simulink model "simcape_real_time_V2"  (R2022b)
settings: Solver=ode8  StartTime=0.0  StopTime=100  FixedStep=0.002  RelTol=1e-3
undefined symbols (not defined in the file): drone_leg, K_LQR, K_LQR_GOC, pitch_init, roll_init, v_pitch_init, v_roll_init, v_x_init, v_y_init, v_yaw_init, v_z_init, X, x_init, Y, y_init, yaw_init, Z, z_init
libraries: sm_lib x55, nesl_utility x12, simulink x7
(part 1 of 3)
settings Model: Creator=tridu  LastModifiedBy=tanda

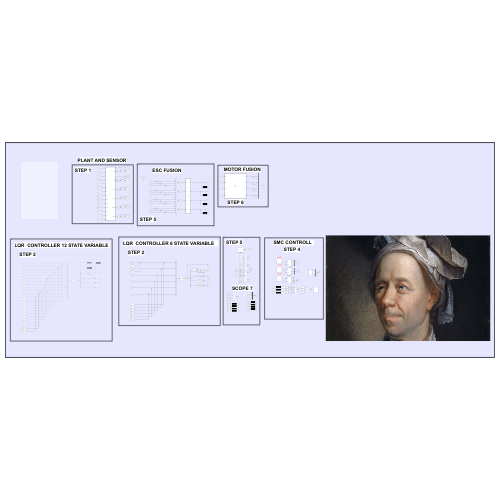
[thumbnail: Simulink's stored preview of the top-level diagram]
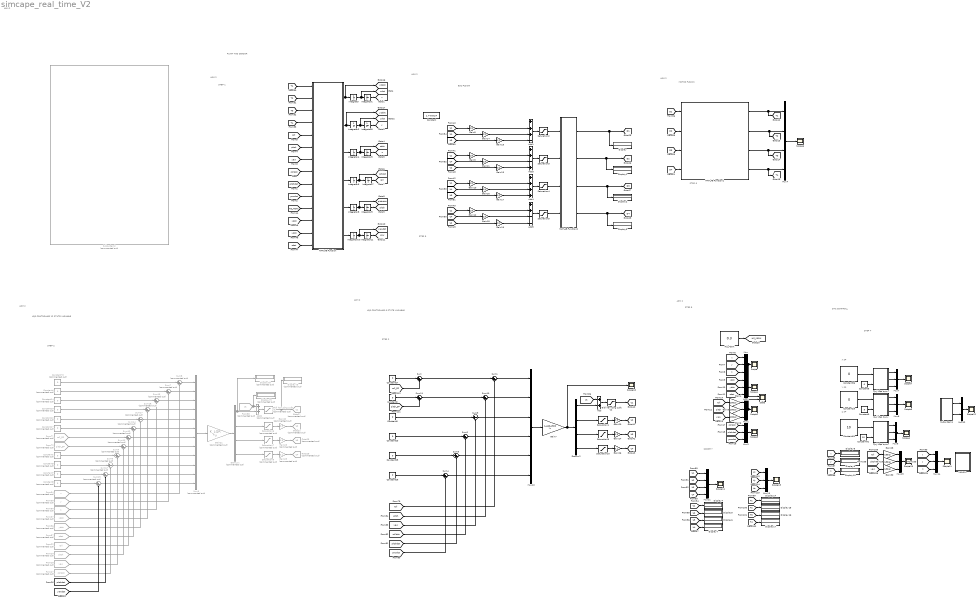
== system simcape_real_time_V2 ==
  note: ARM 2
  note: STEP 5
  note: SCOPE 7
  note: ARM 2
  note: STEP 5
  note: STEP 1
  note: ARM 2
  note: STEP 6
  note: PLANT AND SENSOR
  note: LQR CONTROLLER 12 STATE VARIABLE
  note: STEP 2
  note: ARM 2
  note: STEP 4
  note: X SP
  note: MOTOR FUSION
  note: ARM 2
  note: STEP 2
  note: Y SP
  note: ARM 2
  note: ESC FUSION
  note: Z SP
  note: SMC CONTROLL
  note: ARM 2
  note: LQR CONTROLLER 6 STATE VARIABLE
  Add : Sum
  Add1 : Sum  Inputs=+++-
  Add2 : Sum  Commented=on
  Add3 : Sum  Inputs=++-+
  Add4 : Sum  Inputs=++++
  Add5 : Sum  Inputs=++--
  Constant : Constant  Value=1.7*9.81/4
  Constant{1,4..5,7..8,13..17} (10 alike) : Constant  Commented=on  Value=0
  Constant{2..3,6,23,25..27,29,36} (9 alike) : Constant  Value=0
  Constant31 : Constant  Value=10
  Constant42 : Constant  Value=10
  Constant9 : Constant  Value=5
  Demux1 : Demux  Commented=on
  Demux2 : Demux
  Display{,1..10,14..17} (15 alike) : Display
  Display13 : Display  Commented=on
  Display18 : Display  Commented=on
  Display19 : Display  Commented=on
  From22 : From  Commented=on  GotoTag=roll  TagVisibility=global
  From27 : From  Commented=on  GotoTag=rolldot  TagVisibility=global
  From28 : From  Commented=on  GotoTag=yaw  TagVisibility=global
  From29 : From  Commented=on  GotoTag=pitch  TagVisibility=global
  From34 : From  Commented=on  GotoTag=x  TagVisibility=global
  From35 : From  Commented=on  GotoTag=y  TagVisibility=global
  From36 : From  Commented=on  GotoTag=ydot  TagVisibility=global
  From37 : From  Commented=on  GotoTag=xdot  TagVisibility=global
  From38 : From  Commented=on  GotoTag=Uz  TagVisibility=global
  From57 : From  Commented=on  GotoTag=zdot  TagVisibility=global
  From60 : From  Commented=on  GotoTag=z  TagVisibility=global
  From71 : From  Commented=on  GotoTag=roll_SP  TagVisibility=global
  From72 : From  Commented=on  GotoTag=pitch_SP  TagVisibility=global
  Gain{8..12,14,16,18} (8 alike) : Gain  Gain=1/4
  Gain{13,15,17,19} (4 alike) : Gain  Gain=1/2
  Gain20 : Gain  Gain=0.3
  Gain21 : Gain  Commented=on  Gain=K_LQR  Multiplication=Matrix(K*u)
  Gain22 : Gain  Commented=on  Gain=0.3
  Gain23 : Gain  Commented=on  Gain=0.3
  Gain24 : Gain  Gain=0.3
  Gain25 : Gain  Commented=on  Gain=0.1
  Gain26 : Gain  Gain=0.1
  Gain{4..6,28..30} (6 alike) : Gain  Gain=180/pi
  Gain7 : Gain  Gain=K_LQR_GOC  Multiplication=Matrix(K*u)
  Giới hạn công suất U1 : Saturate  Commented=on  UpperLimit=29.3230*0.3  LowerLimit=-1.7*9.81
  Giới hạn công suất U2 : Saturate  UpperLimit=25  LowerLimit=-1.7*9.81
  Goto21 : Goto  Commented=on  GotoTag=U1  TagVisibility=global
  Goto22 : Goto  Commented=on  GotoTag=U2  TagVisibility=global
  Goto23 : Goto  Commented=on  GotoTag=U3  TagVisibility=global
  Goto29 : Goto  Commented=on  GotoTag=U4  TagVisibility=global
  HS_MSKK : Constant  Value=0.3
  Integrator : Integrator  InitialCondition=v_x_init
  Integrator1 : Integrator  InitialCondition=x_init
  Integrator10 : Integrator  InitialCondition=v_yaw_init
  Integrator11 : Integrator  InitialCondition=yaw_init
  Integrator2 : Integrator  InitialCondition=v_y_init
  Integrator3 : Integrator  InitialCondition=y_init
  Integrator4 : Integrator  InitialCondition=z_init
  Integrator5 : Integrator  InitialCondition=v_z_init
  Integrator6 : Integrator  InitialCondition=v_roll_init
  Integrator7 : Integrator  InitialCondition=roll_init
  Integrator8 : Integrator  InitialCondition=v_pitch_init
  Integrator9 : Integrator  InitialCondition=pitch_init
  MATLAB Function : MATLAB Function  TreatAsAtomicUnit=on
  MATLAB Function1 : MATLAB Function  TreatAsAtomicUnit=on
  MATLAB Function2 : MATLAB Function  TreatAsAtomicUnit=on
  MOVE L : Subsystem
  Mux{,1..3,6..8,13..15} (10 alike) : Mux  Inputs=3
  Mux10 : Mux  Inputs=6
  Mux11 : Mux
  Mux12 : Mux  Inputs=2
  Mux4 : Mux
  Mux5 : Mux  Commented=on  Inputs=12
  Quỹ đạo trục x : Subsystem
  Quỹ đạo trục y : Subsystem
  Quỹ đạo trục z : Subsystem
  Saturation1 : Saturate  UpperLimit=11.5  LowerLimit=-11.5
  Saturation10 : Saturate  UpperLimit=11.5+11.5  LowerLimit=-23
  Saturation{2..5} (4 alike) : Saturate  UpperLimit=11.5  LowerLimit=0
  Saturation6 : Saturate  Commented=on  UpperLimit=11.5  LowerLimit=-11.5
  Saturation7 : Saturate  Commented=on  UpperLimit=11.5  LowerLimit=-11.5
  Saturation8 : Saturate  UpperLimit=11.5  LowerLimit=-11.5
  Saturation9 : Saturate  Commented=on  UpperLimit=11.5  LowerLimit=-11.5
  Scope{,1..4,6..8,10..15} (14 alike) : Scope
  State : Scope  NumInputPorts=2
  Subsystem2 : Subsystem  Commented=on
  Subsystem4 : Subsystem
  Sum : Sum  Inputs=|++
  Sum{1..4,9..10} (6 alike) : Sum  Inputs=|+-
  Sum11 : Sum  Inputs=|++
  Sum{5..8,12..19} (12 alike) : Sum  Commented=on  Inputs=|+-
  tag scope: D1=global, D2=global, D3=global, D4=global, HS_MSKK=global, T1=global, T2=global, T3=global, T4=global, U1=global, U2=global, U3=global, U4=global, pitch=global, pitchdot=global, roll=global, rolldot=global, x2dot=global, x=global, xdot=global, y2dot=global, y=global, yaw=global, yawdot=global, ydot=global, z=global, zdot=global
  wires:
  [pitchdot] -> Mux3/2
  MATLAB Function/3(z2dot) -> Integrator4/1
  Integrator3/1 -> [y]
  Integrator4/1 -> [zdot], Integrator5/1
  Mux1/1 -> Scope1/1
  Integrator7/1 -> [roll]
  [pitchdot] -> MATLAB Function/9(pitch_dot)
  [T3] -> MATLAB Function/3(T3)
  Add5/1 -> Saturation5/1
  MATLAB Function/2(y2dot) -> [y2dot], Integrator2/1
  Mux7/1 -> Scope7/1
  [roll] -> Sum1/2
  [ydot] -> MATLAB Function/13(y_dot)
  Subsystem4/2(Pitch SP) -> Mux12/2
  MATLAB Function1/1(T1) -> Mux4/1, [T1]
  Gain15/1 -> Add1/4
  [roll] -> MATLAB Function/5(roll)
  Mux8/1 -> Scope8/1
  [rolldot] -> Mux3/1
  Integrator11/1 -> [yaw]
  Gain10/1 -> Add4/2
  Giới hạn công suất U2/1 -> [U1]
  Sum2/1 -> Mux10/4
  Mux6/1 -> Scope4/1
  Quỹ đạo trục y/1(X_y) -> Mux8/1
  Quỹ đạo trục z/1(X_z) -> Mux6/1
  Quỹ đạo trục z/2(V_z) -> Mux6/2
  Constant9/1 -> Quỹ đạo trục y/2(v_qd_y)
  Add/1 -> Giới hạn công suất U2/1
  Quỹ đạo trục z/3(A_z) -> Mux6/3
  [HS_MSKK] -> MATLAB Function/11(HS_MSKK)
  Subsystem4/1(Roll SP) -> Mux12/1
  Quỹ đạo trục x/1(X_x) -> Mux7/1
  [pitch_SP] -> Sum11/2
  Mux15/1 -> Scope15/1
  Mux14/1 -> Scope14/1
  [T3] -> Display16/1
  Mux11/1 -> Scope11/1
  [U4] -> Gain16/1
  Integrator9/1 -> [pitch]
  [y] -> Mux14/2
  [U1] -> Gain12/1
  Gain5/1 -> Mux2/2
  Sum17/1 -> Mux5/5
  Quỹ đạo trục x/3(A_x) -> Mux7/3
  [U1] -> Gain8/1
  Gain25/1 -> Goto29/1
  Gain24/1 -> [U3]
  [rolldot] -> Sum2/2
  Integrator8/1 -> [pitchdot], Integrator9/1
  Quỹ đạo trục y/3(A_y) -> Mux8/3
  Mux2/1 -> State/2, Scope2/1
  [pitch] -> Sum10/2
  [zdot] -> Mux1/3
  Constant13/1 -> Sum8/1
  [pitch] -> Gain29/1
  [yaw] -> Gain30/1
  Gain12/1 -> Add5/2
  Demux2/2 -> Saturation1/1
  [yawdot] -> Sum4/2
  Sum14/1 -> Mux5/6
  Gain30/1 -> Mux15/3
  [Ux] -> Mux13/1
  [z] -> Mux14/3
  Mux13/1 -> Scope13/1
  MATLAB Function2/3(D3) -> Display2/1, [D3]
  Sum11/1 -> Sum10/1
  [T4] -> Display17/1
  [yaw] -> Sum9/2
  [roll_SP] -> Sum/2
  Mux10/1 -> Gain7/1
  [x] -> Display8/1
  [D3] -> MATLAB Function1/3(D3)
  Gain20/1 -> [U2]
  [T2] -> Display15/1
  [zdot] -> MATLAB Function/14(z_dot)
  Quỹ đạo trục y/2(V_y) -> Mux8/2
  [Uz] -> Add/1
  [T1] -> Display14/1
  Integrator5/1 -> [z]
  [U3] -> Display6/1
  Giới hạn công suất U1/1 -> Display13/1, Goto21/1
  [D4] -> MATLAB Function1/4(D4)
  [U1] -> Display4/1
  Sum4/1 -> Mux10/6
  [yaw] -> MATLAB Function/7(yaw)
  Gain9/1 -> Add3/2
  Gain4/1 -> Mux2/1
  [U3] -> Mux11/3
  [U1] -> Mux11/1
  [x] -> Mux14/1
  [U2] -> Mux11/2
  MATLAB Function/5(pitch2dot) -> Integrator8/1
  [pitch] -> Gain5/1
  Mux5/1 -> Gain21/1
  [U1] -> Gain9/1
  [Uz] -> Mux13/3
  [U4] -> Gain11/1
  Gain8/1 -> Add1/2
  Gain23/1 -> Goto23/1
  Sum10/1 -> Mux10/2
  Sum9/1 -> Mux10/3
  Gain17/1 -> Add4/4
  Gain6/1 -> Mux2/3
  Integrator10/1 -> [yawdot], Integrator11/1
  Demux1/3 -> Saturation7/1
  Sum3/1 -> Mux10/5
  Mux3/1 -> Scope3/1
  Gain7/1 -> Demux2/1, Scope10/1
  Constant26/1 -> Sum4/1
  [pitch] -> MATLAB Function/6(pitch)
  [U4] -> Mux11/4
  Constant23/1 -> Sum2/1
  Sum15/1 -> Mux5/7
  Constant4/1 -> Sum7/1
  Integrator2/1 -> [ydot], Integrator3/1
  [xdot] -> Mux1/1
  [U2] -> Gain13/1
  [U1] -> Gain10/1
  Quỹ đạo trục x/2(V_x) -> Mux7/2
  Add3/1 -> Saturation3/1
  [xdot] -> MATLAB Function/12(x_dot)
  Add1/1 -> Saturation2/1
  [T1] -> MATLAB Function/1(T1)
  [y] -> Mux/2
  Constant25/1 -> Sum3/1
  Constant6/1 -> Quỹ đạo trục x/2(v_qd_x)
  Mux/1 -> State/1, Scope/1
  Saturation1/1 -> Gain20/1
  [yawdot] -> Mux3/3
  [T4] -> MATLAB Function/4(T4)
  [yawdot] -> MATLAB Function/10(yaw_dot)
  [Uy] -> Mux13/2
  Gain26/1 -> [U4]
  MATLAB Function/1(x2dot) -> [x2dot], Integrator/1
  Saturation3/1 -> MATLAB Function2/2(T2)
  Demux2/3 -> Saturation8/1
  Demux2/4 -> Saturation10/1
  [pitchdot] -> Sum3/2
  Mux12/1 -> Scope12/1
  Gain28/1 -> Mux15/1
  [T2] -> MATLAB Function/2(T2)
  Constant3/1 -> Sum9/1
  Sum1/1 -> Mux10/1
  Sum8/1 -> Mux5/1
  Saturation5/1 -> MATLAB Function2/4(T4)
  [D1] -> MATLAB Function1/1(D1)
  [D2] -> MATLAB Function1/2(D2)
  [z] -> Display10/1
  MATLAB Function1/4(T4) -> Mux4/4, [T4]
  Gain14/1 -> Add1/3
  Constant2/1 -> Sum11/1
  HS_MSKK/1 -> [HS_MSKK]
  MATLAB Function1/2(T2) -> Mux4/2, [T2]
  [U3] -> Gain15/1
  Gain13/1 -> Add3/4
  Gain22/1 -> Goto22/1
  Saturation6/1 -> Gain22/1
  MATLAB Function/6(yaw2dot) -> Integrator10/1
  Gain29/1 -> Mux15/2
  MATLAB Function2/1(D1) -> Display/1, [D1]
  Demux2/1 -> Add/2
  [z] -> Mux/3
  Demux1/2 -> Saturation6/1
  Sum18/1 -> Mux5/4
  Demux1/4 -> Saturation9/1
  MATLAB Function2/2(D2) -> Display1/1, [D2]
  MATLAB Function2/4(D4) -> Display3/1, [D4]
  Saturation2/1 -> MATLAB Function2/1(T1)
  Saturation4/1 -> MATLAB Function2/3(T3)
  Sum/1 -> Sum1/1
  Saturation10/1 -> Gain26/1
  Mux4/1 -> Scope6/1
  Sum13/1 -> Mux5/3
  Sum7/1 -> Mux5/2
  Saturation9/1 -> Gain25/1
  Gain16/1 -> Add4/3
  Add4/1 -> Saturation4/1
  Gain11/1 -> Add3/3
  [roll] -> Gain28/1
  [yaw] -> Gain6/1
  Saturation7/1 -> Gain23/1
  Gain19/1 -> Add5/4
  [U4] -> Display7/1
  Constant42/1 -> Quỹ đạo trục z/2(v_qd_z)
  [U3] -> Gain17/1
  Integrator6/1 -> [rolldot], Integrator7/1
  [y] -> Display9/1
  [ydot] -> Mux1/2
  Constant27/1 -> Sum/1
  [U4] -> Gain18/1
  Sum16/1 -> Mux5/8
  Integrator/1 -> [xdot], Integrator1/1
  [U2] -> Display5/1
  MATLAB Function/4(roll2dot) -> Integrator6/1
  [roll] -> Gain4/1
  MATLAB Function1/3(T3) -> Mux4/3, [T3]
  [U2] -> Gain19/1
  [U4] -> Gain14/1
  Gain18/1 -> Add5/3
  [rolldot] -> MATLAB Function/8(roll_dot)
  Saturation8/1 -> Gain24/1
  Integrator1/1 -> [x]
  [x] -> Mux/1
  Constant36/1 -> Quỹ đạo trục x/1(qf_x)
  Constant31/1 -> Quỹ đạo trục z/1(qf_z)
  Constant29/1 -> Quỹ đạo trục y/1(qf_y)
  Constant1/1 -> Sum5/1
  Sum5/1 -> Mux5/9
  Constant5/1 -> Sum6/1
  Sum6/1 -> Mux5/10
  Constant7/1 -> Sum12/1
  Sum12/1 -> Mux5/11
  Constant8/1 -> Sum19/1
  Sum19/1 -> Mux5/12
  Constant14/1 -> Sum13/1
  Constant15/1 -> Sum18/1
  Constant17/1 -> Sum14/1
  Constant16/1 -> Sum17/1
  From72/1 -> Sum16/1
  From71/1 -> Sum15/1
  From34/1 -> Sum8/2
  From35/1 -> Sum7/2
  From60/1 -> Sum13/2
  From37/1 -> Sum18/2
  From36/1 -> Sum17/2
  From57/1 -> Sum14/2
  From22/1 -> Sum15/2
  From29/1 -> Sum16/2
  From28/1 -> Sum5/2
  From27/1 -> Sum6/2
  [pitchdot] -> Sum12/2
  [yawdot] -> Sum19/2
  Gain21/1 -> Demux1/1
  Demux1/1 -> Add2/2, Display18/1
  Add2/1 -> Giới hạn công suất U1/1
  From38/1 -> Display19/1, Add2/1

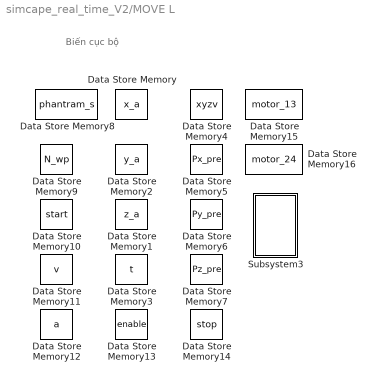
== system simcape_real_time_V2/MOVE L ==
  note: Biến cục bộ
  Data Store Memory : DataStoreMemory  DataStoreName=x_a  WriteAfterWriteMsg=warning  ShowAdditionalParam=off
  Data Store Memory1 : DataStoreMemory  DataStoreName=z_a  WriteAfterWriteMsg=warning  ShowAdditionalParam=off
  Data Store Memory10 : DataStoreMemory  DataStoreName=start  WriteAfterWriteMsg=warning  ShowAdditionalParam=off
  Data Store Memory11 : DataStoreMemory  DataStoreName=v  WriteAfterWriteMsg=warning  ShowAdditionalParam=off
  Data Store Memory12 : DataStoreMemory  DataStoreName=a  WriteAfterWriteMsg=warning  ShowAdditionalParam=off
  Data Store Memory13 : DataStoreMemory  DataStoreName=enable  WriteAfterWriteMsg=warning  ShowAdditionalParam=off
  Data Store Memory14 : DataStoreMemory  DataStoreName=stop  WriteAfterWriteMsg=warning  ShowAdditionalParam=off
  Data Store Memory15 : DataStoreMemory  DataStoreName=motor_13  WriteAfterWriteMsg=warning  ShowAdditionalParam=off  OutDataTypeStr=double  Dimensions=1
  Data Store Memory16 : DataStoreMemory  DataStoreName=motor_24  WriteAfterWriteMsg=warning  ShowAdditionalParam=off  OutDataTypeStr=double  Dimensions=1
  Data Store Memory2 : DataStoreMemory  DataStoreName=y_a  WriteAfterWriteMsg=warning  ShowAdditionalParam=off
  Data Store Memory3 : DataStoreMemory  DataStoreName=t  WriteAfterWriteMsg=warning  ShowAdditionalParam=off
  Data Store Memory4 : DataStoreMemory  DataStoreName=xyzv  WriteAfterWriteMsg=warning  ShowAdditionalParam=off  OutDataTypeStr=double  Dimensions=4
  Data Store Memory5 : DataStoreMemory  DataStoreName=Px_pre  WriteAfterWriteMsg=warning  ShowAdditionalParam=off
  Data Store Memory6 : DataStoreMemory  DataStoreName=Py_pre  WriteAfterWriteMsg=warning  ShowAdditionalParam=off
  Data Store Memory7 : DataStoreMemory  DataStoreName=Pz_pre  WriteAfterWriteMsg=warning  ShowAdditionalParam=off
  Data Store Memory8 : DataStoreMemory  DataStoreName=phantram_s  WriteAfterWriteMsg=warning  ShowAdditionalParam=off
  Data Store Memory9 : DataStoreMemory  DataStoreName=N_wp  WriteAfterWriteMsg=warning  ShowAdditionalParam=off
  Subsystem3 : Subsystem

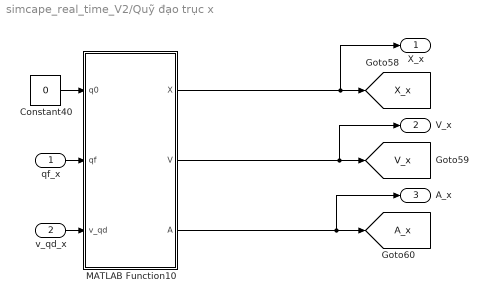
== system simcape_real_time_V2/Quỹ đạo trục x ==
  qf_x : Inport
  v_qd_x : Inport  Port=2
  Constant40 : Constant  Value=0
  MATLAB Function10 : MATLAB Function  TreatAsAtomicUnit=on
  X_x : Outport
  V_x : Outport  Port=2
  A_x : Outport  Port=3
  tag scope: A_x=global, V_x=global, X_x=global
  wires:
  Constant40/1 -> MATLAB Function10/1(q0)
  v_qd_x/1 -> MATLAB Function10/3(v_qd)
  qf_x/1 -> MATLAB Function10/2(qf)
  MATLAB Function10/1(X) -> [X_x], X_x/1
  MATLAB Function10/3(A) -> [A_x], A_x/1
  MATLAB Function10/2(V) -> [V_x], V_x/1

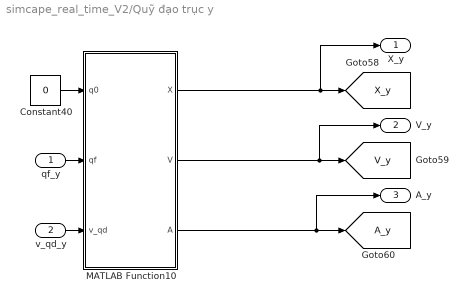
== system simcape_real_time_V2/Quỹ đạo trục y ==
  qf_y : Inport
  v_qd_y : Inport  Port=2
  Constant40 : Constant  Value=0
  MATLAB Function10 : MATLAB Function  TreatAsAtomicUnit=on
  X_y : Outport
  V_y : Outport  Port=2
  A_y : Outport  Port=3
  tag scope: A_y=global, V_y=global, X_y=global
  wires:
  Constant40/1 -> MATLAB Function10/1(q0)
  v_qd_y/1 -> MATLAB Function10/3(v_qd)
  qf_y/1 -> MATLAB Function10/2(qf)
  MATLAB Function10/1(X) -> [X_y], X_y/1
  MATLAB Function10/2(V) -> [V_y], V_y/1
  MATLAB Function10/3(A) -> A_y/1, [A_y]

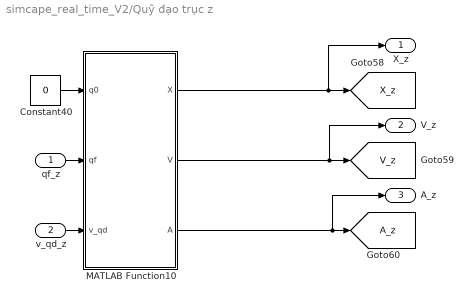
== system simcape_real_time_V2/Quỹ đạo trục z ==
  qf_z : Inport
  v_qd_z : Inport  Port=2
  Constant40 : Constant  Value=0
  MATLAB Function10 : MATLAB Function  TreatAsAtomicUnit=on
  X_z : Outport
  V_z : Outport  Port=2
  A_z : Outport  Port=3
  tag scope: A_z=global, V_z=global, X_z=global
  wires:
  Constant40/1 -> MATLAB Function10/1(q0)
  v_qd_z/1 -> MATLAB Function10/3(v_qd)
  qf_z/1 -> MATLAB Function10/2(qf)
  MATLAB Function10/2(V) -> [V_z], V_z/1
  MATLAB Function10/3(A) -> [A_z], A_z/1
  MATLAB Function10/1(X) -> [X_z], X_z/1
